simulink model "aero421_finalProject"  (R2023a)
settings: Solver=FixedStepAuto  StartTime=0.0  StopTime=tspan  FixedStep=10  RelTol=1e-3
values from neighbouring files (symbols this model uses):
  T = 0    [T.m]
undefined symbols (not defined in the file or in its folder): E_b_ECI_0, J_deploy, q_b_ECI_0, w_b_ECI_0
settings Model: Creator=emehiel  LastModifiedBy=tlunn
settings SolverCC: AlgebraicLoopSolver=TrustRegion
settings DebuggingCC: UnconnectedInputMsg=warning  UnconnectedOutputMsg=warning  UnconnectedLineMsg=warning
settings ModelReferenceCC: EnableRefExpFcnMdlSchedulingChecks=on

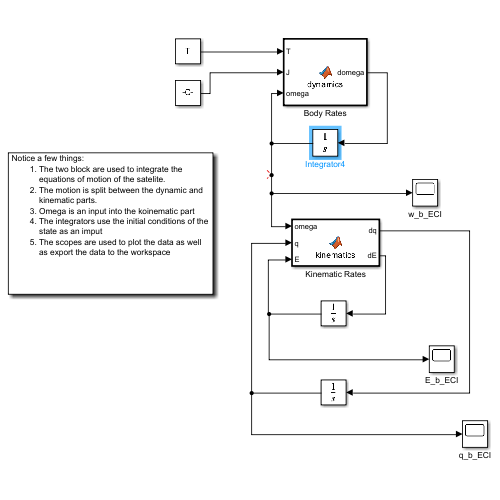
[thumbnail: Simulink's stored preview of the top-level diagram]
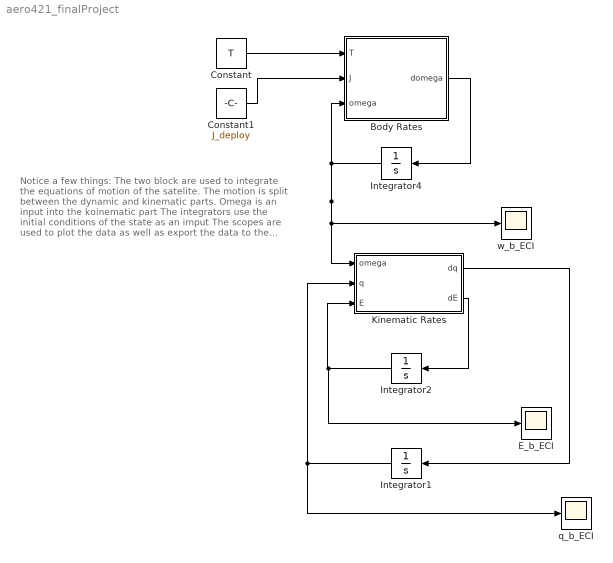
== system aero421_finalProject ==
  note: Notice a few things:
      | The two block are used to integrate the equations of motion of the satelite.
      | The motion is split between the dynamic and kinematic parts.
      | Omega is an input into the koinematic part
      | The integrators use the initial conditions of the state as an imput
      | The scopes are used to plot the data as well as export the data to the workspace
  Body Rates : MATLAB Function  TreatAsAtomicUnit=on
  Constant : Constant  Value=T
  Constant1 : Constant  Value=J_deploy
  E_b_ECI : Scope
  Integrator1 : Integrator  InitialCondition=q_b_ECI_0
  Integrator2 : Integrator  InitialCondition=E_b_ECI_0
  Integrator4 : Integrator  InitialCondition=w_b_ECI_0
  Kinematic Rates : MATLAB Function  TreatAsAtomicUnit=on
  q_b_ECI : Scope
  w_b_ECI : Scope
  wires:
  Constant/1 -> Body Rates/1(T)
  Constant1/1 -> Body Rates/2(J)
  Body Rates/1(domega) -> Integrator4/1
  Integrator4/1 -> Body Rates/3(omega), Kinematic Rates/1(omega), w_b_ECI/1
  Integrator2/1 -> E_b_ECI/1, Kinematic Rates/3(E)
  Integrator1/1 -> q_b_ECI/1, Kinematic Rates/2(q)
  Kinematic Rates/2(dE) -> Integrator2/1
  Kinematic Rates/1(dq) -> Integrator1/1

== matlab function aero421_finalProject/Kinematic Rates ==
  data: omega input; q input; dq output; E input; dE output
function [dq,dE] = kinematics(omega, q, E)
%#codegen

% unpack quaternion

% compute the derivative of the quaternion components here

% compute the derivative of the Euler Angle components here

== matlab function aero421_finalProject/Body Rates ==
  data: T input; J input; omega input; domega output
function domega = dynamics(T, J, omega)
%#codegen

% Compute the derivative of the angular velocity $\omega$ here

% deployed moment of inertia for sensor, in kg*m^2
Jx_sensor = 1/12*sensor_mass*(sensor_base^2+sensor_thick^2)+sensor_mass*(bus_side/2+sensor_height/2)^2; % Moment of Inertia of Sensor about x axis, m^4
Jy_sensor = Jx_sensor;
Jz_sensor = 1/12*sensor_mass*(sensor_base^2+sensor_thick^2);

% deployed moment of inertia for each solar panel, in kg*m^2
Jx_solar = 1/12*solar_mass*(solar_base^2+solar_thick^2)+solar_mass*(bus_side/2+solar_base/2)^2;
Jy_solar = 1/12*solar_mass*(solar_height^2+solar_thick^2);
Jz_solar = 1/12*solar_mass*(solar_height^2+solar_base^2)+solar_mass*(bus_side/2+solar_base/2)^2;

% deployed moment of inertia for bus, in kg*m^2
Jx_bus = 1/12*bus_mass*(2*bus_side^2);
Jy_bus = Jx_bus;
Jz_bus = Jx_bus;

%moment of inertia for deployed configuration, in kg*m^2
Jx_deploy = Jx_sensor+2*Jx_solar+Jx_bus;
Jy_deploy = Jy_sensor+2*Jy_solar+Jy_bus;
Jz_deploy = Jz_sensor+2*Jz_solar+Jz_bus;
J_deploy = [Jx_deploy 0 0 
            0 Jy_deploy 0
            0 0 Jz_deploy];

J = J_deploy;

T = 0;

w_b_ECI_deploy = [0.001; -0.001; 0.002];
